simulink model "Modelo_final"  (R2020a)
settings: Solver=VariableStepAuto  StartTime=0.0  StopTime=20  RelTol=1e-3
values from neighbouring files (symbols this model uses):
  ba = Jeq*n*wpos    (= 0.0113019895361)    [Parametros.m]
  beq = bm+(bl/r^2)    (= 1.5e-05)    [Parametros.m]
  Cts = 1.091    [Parametros.m]
  Jeq = Jm+(Jl/r^2)    (= 5.65099476805e-06)    [Parametros.m]
  ke_omega = 3200^2    (= 10240000)    [Parametros.m]
  ke_thetha = 6400    [Parametros.m]
  ksa = Jeq*n*wpos^2    (= 9.04159162887)    [Parametros.m]
  ksia = Jeq*wpos^3    (= 2893.30932124)    [Parametros.m]
  lambdam = .01546    (= 0.01546)    [Parametros.m]
  Ld = 6.6e-3    (= 0.0066)    [Parametros.m]
  Lls = 0.8e-3    (= 0.0008)    [Parametros.m]
  Lq = 5.8e-3    (= 0.0058)    [Parametros.m]
  Pp = 3    [Parametros.m]
  r = 314.3008    [Parametros.m]
  R0p = 4    [Parametros.m]
  Rdp = 33    [Parametros.m]
  Rqp = 29    [Parametros.m]
  Rs = 1.02    [Parametros.m]
  Rs40 = 1.02    [Parametros.m]
  Rts = 55    [Parametros.m]
undefined symbols (not defined in the file or in its folder): sigbuilder_block
settings Model: Creator=tinsu  LastModifiedBy=tinsu

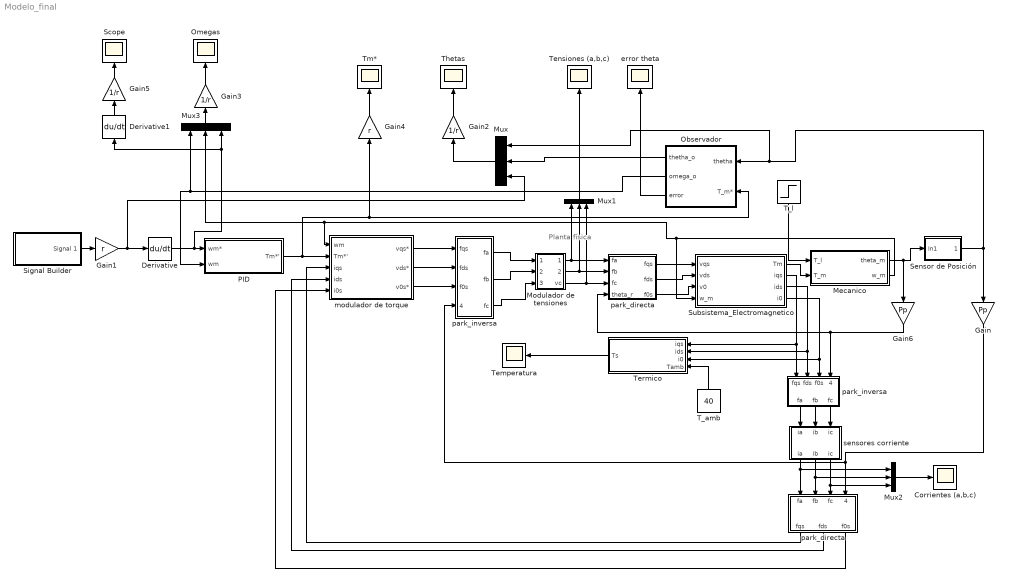
== system Modelo_final ==
  note: Planta física
  Corrientes (a,b,c) : Scope
  Derivative : Derivative
  Derivative1 : Derivative
  Gain : Gain  Gain=Pp
  Gain1 : Gain  Gain=r
  Gain2 : Gain  Gain=1/r
  Gain3 : Gain  Gain=1/r
  Gain4 : Gain  Gain=r
  Gain5 : Gain  Gain=1/r
  Gain6 : Gain  Gain=Pp
  Mecanico : Subsystem
  Modulador de tensiones : Subsystem
  Mux{,1..3} (4 alike) : Mux  Inputs=3
  Observador : Subsystem
  Omegas : Scope
  PID : Subsystem
  Scope : Scope
  Sensor de Posición : Subsystem
  Signal Builder : Subsystem  Tag=STV Subsys  LoadFcn=sigbuilder_block('load');  StartFcn=sigbuilder_block('start');  StopFcn=sigbuilder_block('stop');  ClipboardFcn=sigbuilder_block('clipboard');  mask(Sigbuilder block){tuvar=[0:10]}
      mask help: Simulink:masks:SigbuilderBlock_MD
      mask init:
      | if ~strcmp(get_param(bdroot(gcbh),'SimulationStatus'),'stopped') tuvar = sigbuilder_block('maskInit'); end
      settings: CopyFcn=sigbuilder_block('copy');  DeleteFcn=sigbuilder_block('delete');  ModelCloseFcn=sigbuilder_block('modelClose');  PreSaveFcn=sigbuilder_block('preSave');  PauseFcn=sigbuilder_block('pause');  ContinueFcn=sigbuilder_block('continue');  NameChangeFcn=sigbuilder_block('namechange');  OpenFcn=sigbuilder_block('open',[437.6 199.2 550.4 400 ]);  CloseFcn=sigbuilder_block('close');
      mask Display: plot(0, 0, 100, 100,[2, 2, 32, 32, 2], [68, 8, 8, 68, 68],[32, 2], [38, 38], [32, 19, 2],[53, 60, 44], [32, 17, 17, 2],[16, 16, 31, 31]);txt = getActiveGroup(gcbh);text(2, 100, txt,'verticalAlignment', 'top');
  Subsistema_Electromagnetico : Subsystem
  T_amb : Constant  Value=40
  T_l : Step  After=1.57  SampleTime=0
  Temperatura : Scope
  Tensiones (a,b,c) : Scope
  Termico : Subsystem
  Thetas : Scope
  Tm* : Scope
  error theta : Scope
  modulador de torque : Subsystem
  park_directa : Subsystem
  "park_directa " : Subsystem
  park_inversa : Subsystem
  "park_inversa " : Subsystem
  sensores corriente : Subsystem
  wires:
  Mux3/1 -> Gain3/1
  "park_directa "/2(fds) -> modulador de torque/4(ids)
  Gain3/1 -> Omegas/1
  Modulador de tensiones/1(va) -> Mux1/1, park_directa/1("fa ")
  Signal Builder/1(Signal 1) -> Gain1/1
  Gain4/1 -> Tm*/1
  Termico/1(Ts) -> Temperatura/1
  sensores corriente/1("ia ") -> "park_directa "/1("fa "), Mux2/1
  Observador/3(error) -> error theta/1
  Gain/1 -> "park_directa "/4(theta_r1), park_inversa/4(theta_r)
  "park_inversa "/1(fa) -> sensores corriente/1(ia)
  "park_directa "/1(fqs) -> modulador de torque/3(iqs)
  Mux1/1 -> Tensiones (a,b,c)/1
  Mux/1 -> Gain2/1
  Gain1/1 -> Derivative/1, Mux/3
  T_l/1 -> Mecanico/1(T_l)
  sensores corriente/2("ib ") -> "park_directa "/2("fb "), Mux2/2
  Mux2/1 -> Corrientes (a,b,c)/1
  park_directa/2(fds) -> Subsistema_Electromagnetico/2(vds)
  Gain2/1 -> Thetas/1
  Observador/1(thetha_o) -> Mux/2
  Mecanico/2(w_m) -> modulador de torque/1(wm), Mux3/2, Subsistema_Electromagnetico/4(w_m)
  park_directa/3(f0s) -> Subsistema_Electromagnetico/3(v0)
  Subsistema_Electromagnetico/2(iqs) -> Termico/1(iqs), "park_inversa "/1(fqs)
  Subsistema_Electromagnetico/3(ids) -> "park_inversa "/2(fds), Termico/2(ids)
  Observador/2(omega_o) -> Mux3/1, PID/2(wm)
  sensores corriente/3("ic ") -> Mux2/3, "park_directa "/3("fc ")
  Subsistema_Electromagnetico/4(i0) -> Termico/3(i0), "park_inversa "/3(f0s)
  Subsistema_Electromagnetico/1(Tm) -> Mecanico/2(T_m)
  "park_inversa "/2(fb) -> sensores corriente/2(ib)
  "park_inversa "/3(fc) -> sensores corriente/3(ic)
  Mecanico/1(theta_m) -> Gain6/1, Sensor de Posición/1(In1)
  modulador de torque/2(vds*) -> park_inversa/2(fds)
  PID/1(Tm*') -> Gain4/1, Observador/2(T_m*), modulador de torque/2(Tm*')
  park_inversa/1(fa) -> Modulador de tensiones/1(va*)
  park_inversa/3(fc) -> Modulador de tensiones/3(vc*)
  Modulador de tensiones/3(vc) -> Mux1/3, park_directa/3("fc ")
  "park_directa "/3(f0s) -> modulador de torque/5(i0s)
  modulador de torque/3(v0s*) -> park_inversa/3(f0s)
  park_inversa/2(fb) -> Modulador de tensiones/2(vb*)
  Modulador de tensiones/2(vb) -> Mux1/2, park_directa/2("fb ")
  modulador de torque/1(vqs*) -> park_inversa/1(fqs)
  T_amb/1 -> Termico/4(Tamb)
  park_directa/1(fqs) -> Subsistema_Electromagnetico/1(vqs)
  Derivative/1 -> Derivative1/1, Mux3/3, PID/1(wm*)
  Sensor de Posición/1(Out1) -> Gain/1, Mux/1, Observador/1(thetha)
  Derivative1/1 -> Gain5/1
  Gain5/1 -> Scope/1
  Gain6/1 -> "park_inversa "/4(theta_r), park_directa/4(theta_r)

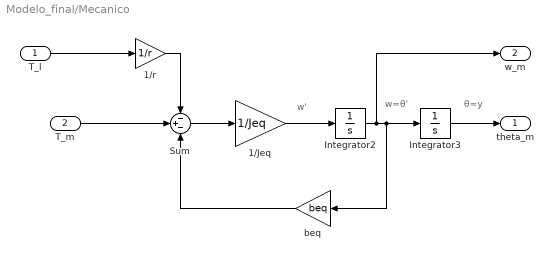
== system Modelo_final/Mecanico ==
  note: w=θ'
  note: θ=y
  note: w'
  T_l : Inport
  T_m : Inport  Port=2
  "1/Jeq " : Gain  Gain=1/Jeq
  "1/r " : Gain  Gain=1/r
  Integrator2 : Integrator
  Integrator3 : Integrator
  Sum : Sum  Inputs=-+-
  "beq " : Gain  Gain=beq
  theta_m : Outport
  w_m : Outport  Port=2
  wires:
  "1/r "/1 -> Sum/1
  "1/Jeq "/1 -> Integrator2/1
  Integrator3/1 -> theta_m/1
  Sum/1 -> "1/Jeq "/1
  "beq "/1 -> Sum/3
  Integrator2/1 -> Integrator3/1, "beq "/1, w_m/1
  T_m/1 -> Sum/2
  T_l/1 -> "1/r "/1

== system Modelo_final/Modulador de tensiones ==
  va* : Inport
  vb* : Inport  Port=2
  vc* : Inport  Port=3
  Gain : Gain
  Gain1 : Gain
  Gain2 : Gain
  va : Outport
  vb : Outport  Port=2
  vc : Outport  Port=3
  wires:
  va*/1 -> Gain/1
  vb*/1 -> Gain1/1
  vc*/1 -> Gain2/1
  Gain/1 -> va/1
  Gain1/1 -> vb/1
  Gain2/1 -> vc/1

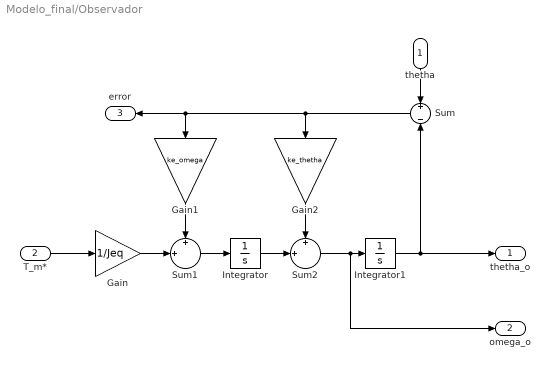
== system Modelo_final/Observador ==
  thetha : Inport
  T_m* : Inport  Port=2
  Gain : Gain  Gain=1/Jeq
  Gain1 : Gain  Gain=ke_omega
  Gain2 : Gain  Gain=ke_thetha
  Integrator : Integrator
  Integrator1 : Integrator
  Sum : Sum  Inputs=+||-
  Sum1 : Sum  Inputs=+|+||
  Sum2 : Sum  Inputs=+|+||
  thetha_o : Outport
  omega_o : Outport  Port=2
  error : Outport  Port=3
  wires:
  Integrator1/1 -> thetha_o/1, Sum/2
  T_m*/1 -> Gain/1
  Sum/1 -> error/1, Gain1/1, Gain2/1
  Gain1/1 -> Sum1/1
  thetha/1 -> Sum/1
  Integrator/1 -> Sum2/2
  Sum1/1 -> Integrator/1
  Gain2/1 -> Sum2/1
  Gain/1 -> Sum1/2
  Sum2/1 -> omega_o/1, Integrator1/1

== system Modelo_final/PID ==
  note: I
  note: e_dtheta_m
  note: e_wm
  note: e_theta_m
  note: P
  note: D
  wm* : Inport
  wm : Inport  Port=2
  Integrator : Integrator
  Integrator1 : Integrator
  Sum : Sum  Inputs=|+-
  Sum1 : Sum  Inputs=|+++
  ba : Gain  Gain=ba
  ksa : Gain  Gain=ksa
  ksia : Gain  Gain=ksia
  Tm*' : Outport
  wires:
  Integrator1/1 -> ksia/1
  Sum1/1 -> Tm*'/1
  wm*/1 -> Sum/1
  ba/1 -> Sum1/3
  Sum/1 -> Integrator/1, ba/1
  ksa/1 -> Sum1/2
  ksia/1 -> Sum1/1
  wm/1 -> Sum/2
  Integrator/1 -> Integrator1/1, ksa/1

== system Modelo_final/Sensor de Posición ==
  In1 : Inport
  Gain : Gain
  Out1 : Outport
  wires:
  In1/1 -> Gain/1
  Gain/1 -> Out1/1

== system Modelo_final/Signal Builder ==
  Demux : Demux  Tag=STV Demux  Outputs=1
      settings: DisplayOption=none
  FromWs : FromWorkspace  Tag=STV FromWs  VariableName=tuvar
      SigBuilderData=|
      | common.afterFinalStr = 'Extrapolate'
      | common.sampleTime = 0
      | dataSet.timeRange = [0 20]
      | dataSet.name = 'Group 1'
      | sbobj.Groups.Name = 'Group 1'
      | sbobj.Groups.Signals.Name = 'Signal 1'
      | sbobj.Groups.Signals.XData = [0 2 7 13 18 20]
      | sbobj.Groups.Signals.YData = [0 0 6.28318530718 6.28318530718 0 0]
      | sbobj.Groups.TimeRange = [0 20]
  Signal 1 : Outport  Tag=STV Outport
  wires:
  Demux/1 -> Signal 1/1
  FromWs/1 -> Demux/1

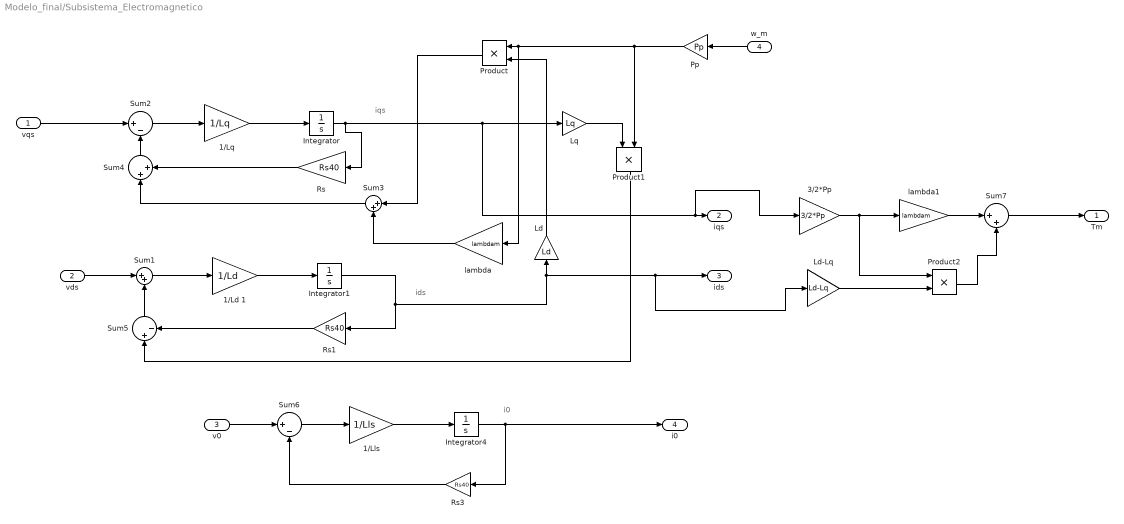
== system Modelo_final/Subsistema_Electromagnetico ==
  note: iqs
  note: i0
  note: ids
  vqs : Inport
  vds : Inport  Port=2
  v0 : Inport  Port=3
  w_m : Inport  Port=4
  1/Ld 1 : Gain  Gain=1/Ld
  1/Lls : Gain  Gain=1/Lls
  "1/Lq " : Gain  Gain=1/Lq
  3/2*Pp : Gain  Gain=3/2*Pp
  Integrator : Integrator
  Integrator1 : Integrator
  Integrator4 : Integrator
  Ld : Gain  Gain=Ld
  Ld-Lq : Gain  Gain=Ld-Lq
  "Lq " : Gain  Gain=Lq
  Pp : Gain  Gain=Pp
  Product : Product
  Product1 : Product
  Product2 : Product
  Rs : Gain  Gain=Rs40
  Rs1 : Gain  Gain=Rs40
  Rs3 : Gain  Gain=Rs40
  Sum{1,3..4,7} (4 alike) : Sum  Inputs=|++
  Sum2 : Sum  Inputs=|+-
  Sum5 : Sum  Inputs=|+-
  Sum6 : Sum  Inputs=|+-
  lambda : Gain  Gain=lambdam
  lambda1 : Gain  Gain=lambdam
  Tm : Outport
  iqs : Outport  Port=2
  ids : Outport  Port=3
  i0 : Outport  Port=4
  wires:
  Integrator4/1 -> i0/1, Rs3/1
  Sum6/1 -> 1/Lls/1
  Sum5/1 -> Sum1/2
  Rs/1 -> Sum4/2
  Sum4/1 -> Sum2/2
  "1/Lq "/1 -> Integrator/1
  Integrator1/1 -> Rs1/1, Ld-Lq/1, ids/1, Ld/1
  Integrator/1 -> Rs/1, 3/2*Pp/1, iqs/1, "Lq "/1
  Rs3/1 -> Sum6/2
  1/Lls/1 -> Integrator4/1
  Product/1 -> Sum3/1
  Pp/1 -> lambda/1, Product/1, Product1/2
  "Lq "/1 -> Product1/1
  Sum1/1 -> 1/Ld 1/1
  Product1/1 -> Sum5/1
  1/Ld 1/1 -> Integrator1/1
  Sum2/1 -> "1/Lq "/1
  v0/1 -> Sum6/1
  lambda/1 -> Sum3/2
  Ld/1 -> Product/2
  Rs1/1 -> Sum5/2
  vds/1 -> Sum1/1
  Sum3/1 -> Sum4/1
  vqs/1 -> Sum2/1
  w_m/1 -> Pp/1
  Ld-Lq/1 -> Product2/2
  lambda1/1 -> Sum7/1
  Product2/1 -> Sum7/2
  3/2*Pp/1 -> Product2/1, lambda1/1
  Sum7/1 -> Tm/1

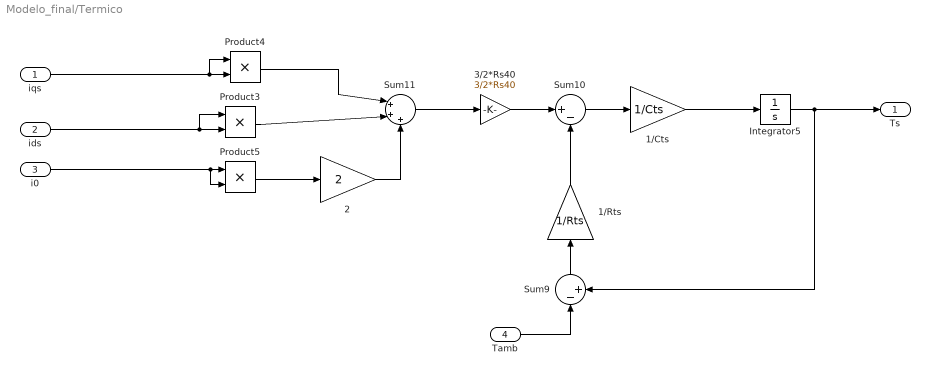
== system Modelo_final/Termico ==
  iqs : Inport
  ids : Inport  Port=2
  i0 : Inport  Port=3
  Tamb : Inport  Port=4
  1/Cts : Gain  Gain=1/Cts
  1/Rts : Gain  Gain=1/Rts
  "2 " : Gain  Gain=2
  "3/2*Rs40 " : Gain  Gain=3/2*Rs40
  Integrator5 : Integrator
  Product3 : Product
  Product4 : Product
  Product5 : Product
  Sum10 : Sum  Inputs=|+-
  Sum11 : Sum  Inputs=|+++
  Sum9 : Sum  Inputs=|-+
  Ts : Outport
  wires:
  "3/2*Rs40 "/1 -> Sum10/1
  1/Cts/1 -> Integrator5/1
  Sum10/1 -> 1/Cts/1
  Tamb/1 -> Sum9/1
  Integrator5/1 -> Ts/1, Sum9/2
  Product3/1 -> Sum11/2
  ids/1 -> Product3/1, Product3/2
  "2 "/1 -> Sum11/3
  Sum11/1 -> "3/2*Rs40 "/1
  Product5/1 -> "2 "/1
  i0/1 -> Product5/2, Product5/1
  1/Rts/1 -> Sum10/2
  Product4/1 -> Sum11/1
  Sum9/1 -> 1/Rts/1
  iqs/1 -> Product4/1, Product4/2

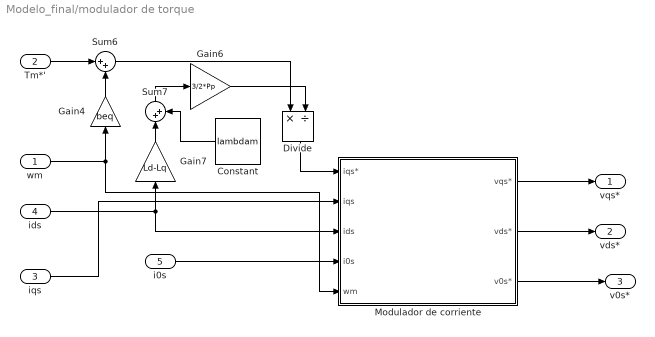
== system Modelo_final/modulador de torque ==
  wm : Inport
  Tm*' : Inport  Port=2
  iqs : Inport  Port=3
  ids : Inport  Port=4
  i0s : Inport  Port=5
  Constant : Constant  Value=lambdam
  Divide : Product  Inputs=*/
  Gain4 : Gain  Gain=beq
  Gain6 : Gain  Gain=3/2*Pp
  Gain7 : Gain  Gain=Ld-Lq
  Modulador de corriente : Subsystem
  Sum6 : Sum  Inputs=|++
  Sum7 : Sum  Inputs=|++
  vqs* : Outport
  vds* : Outport  Port=2
  v0s* : Outport  Port=3
  wires:
  iqs/1 -> Modulador de corriente/2(iqs)
  ids/1 -> Modulador de corriente/3(ids), Gain7/1
  Modulador de corriente/2(vds*) -> vds*/1
  Modulador de corriente/1(vqs*) -> vqs*/1
  Gain7/1 -> Sum7/1
  i0s/1 -> Modulador de corriente/4(i0s)
  Gain6/1 -> Divide/2
  Divide/1 -> Modulador de corriente/1(iqs*)
  wm/1 -> Modulador de corriente/5(wm), Gain4/1
  Gain4/1 -> Sum6/2
  Constant/1 -> Sum7/2
  Tm*'/1 -> Sum6/1
  Sum7/1 -> Gain6/1
  Sum6/1 -> Divide/1
  Modulador de corriente/3(v0s*) -> v0s*/1

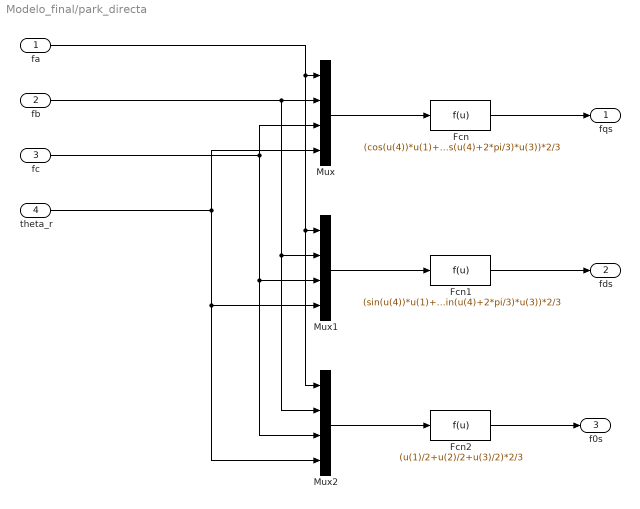
== system Modelo_final/park_directa ==
  "fa " : Inport
  "fb " : Inport  Port=2
  "fc " : Inport  Port=3
  theta_r : Inport  Port=4
  Fcn : Fcn  Expr=(cos(u(4))*u(1)+cos(u(4)-2*pi/3)*u(2)+cos(u(4)+2*pi/3)*u(3))*2/3
  Fcn1 : Fcn  Expr=(sin(u(4))*u(1)+sin(u(4)-2*pi/3)*u(2)+sin(u(4)+2*pi/3)*u(3))*2/3
  Fcn2 : Fcn  Expr=(u(1)/2+u(2)/2+u(3)/2)*2/3
  Mux : Mux
  Mux1 : Mux
  Mux2 : Mux
  fqs : Outport
  fds : Outport  Port=2
  f0s : Outport  Port=3
  wires:
  "fc "/1 -> Mux/3, Mux1/3, Mux2/3
  "fb "/1 -> Mux/2, Mux1/2, Mux2/2
  Fcn/1 -> fqs/1
  Fcn2/1 -> f0s/1
  theta_r/1 -> Mux/4, Mux1/4, Mux2/4
  Mux2/1 -> Fcn2/1
  Mux1/1 -> Fcn1/1
  Mux/1 -> Fcn/1
  Fcn1/1 -> fds/1
  "fa "/1 -> Mux1/1, Mux2/1, Mux/1

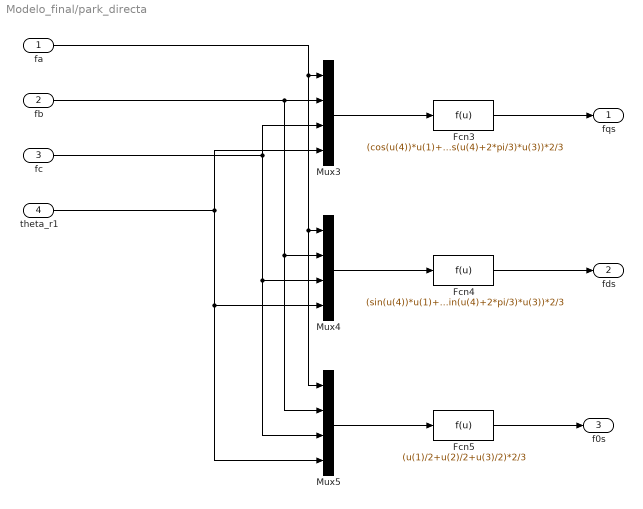
== system Modelo_final/park_directa  ==
  "fa " : Inport
  "fb " : Inport  Port=2
  "fc " : Inport  Port=3
  theta_r1 : Inport  Port=4
  Fcn3 : Fcn  Expr=(cos(u(4))*u(1)+cos(u(4)-2*pi/3)*u(2)+cos(u(4)+2*pi/3)*u(3))*2/3
  Fcn4 : Fcn  Expr=(sin(u(4))*u(1)+sin(u(4)-2*pi/3)*u(2)+sin(u(4)+2*pi/3)*u(3))*2/3
  Fcn5 : Fcn  Expr=(u(1)/2+u(2)/2+u(3)/2)*2/3
  Mux3 : Mux
  Mux4 : Mux
  Mux5 : Mux
  fqs : Outport
  fds : Outport  Port=2
  f0s : Outport  Port=3
  wires:
  Mux5/1 -> Fcn5/1
  "fa "/1 -> Mux4/1, Mux5/1, Mux3/1
  Fcn4/1 -> fds/1
  Mux3/1 -> Fcn3/1
  Mux4/1 -> Fcn4/1
  "fb "/1 -> Mux3/2, Mux4/2, Mux5/2
  Fcn3/1 -> fqs/1
  Fcn5/1 -> f0s/1
  theta_r1/1 -> Mux3/4, Mux4/4, Mux5/4
  "fc "/1 -> Mux3/3, Mux4/3, Mux5/3

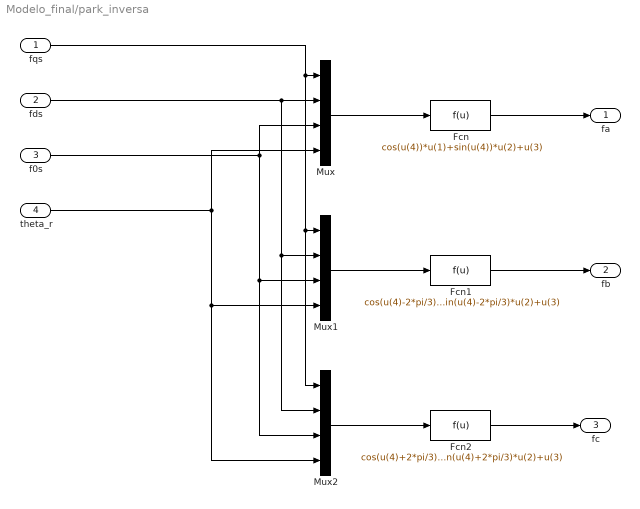
== system Modelo_final/park_inversa ==
  fqs : Inport
  fds : Inport  Port=2
  f0s : Inport  Port=3
  theta_r : Inport  Port=4
  Fcn : Fcn  Expr=cos(u(4))*u(1)+sin(u(4))*u(2)+u(3)
  Fcn1 : Fcn  Expr=cos(u(4)-2*pi/3)*u(1)+sin(u(4)-2*pi/3)*u(2)+u(3)
  Fcn2 : Fcn  Expr=cos(u(4)+2*pi/3)*u(1)+sin(u(4)+2*pi/3)*u(2)+u(3)
  Mux : Mux
  Mux1 : Mux
  Mux2 : Mux
  fa : Outport
  fb : Outport  Port=2
  fc : Outport  Port=3
  wires:
  f0s/1 -> Mux/3, Mux1/3, Mux2/3
  fds/1 -> Mux/2, Mux1/2, Mux2/2
  Fcn/1 -> fa/1
  Fcn2/1 -> fc/1
  theta_r/1 -> Mux/4, Mux1/4, Mux2/4
  Mux2/1 -> Fcn2/1
  Mux1/1 -> Fcn1/1
  Mux/1 -> Fcn/1
  Fcn1/1 -> fb/1
  fqs/1 -> Mux1/1, Mux2/1, Mux/1

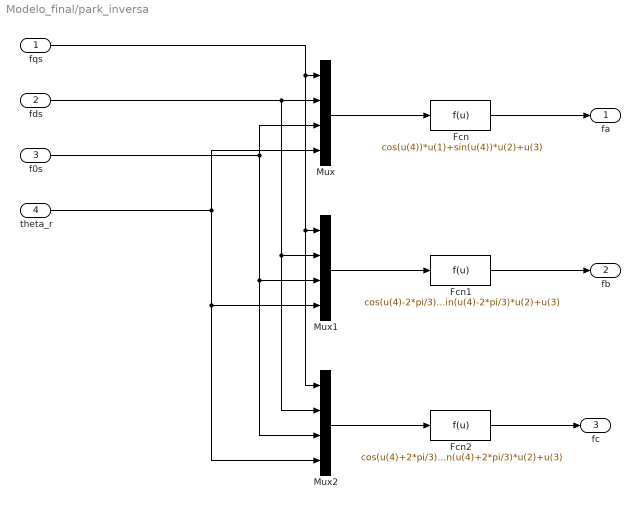
== system Modelo_final/park_inversa  ==
  fqs : Inport
  fds : Inport  Port=2
  f0s : Inport  Port=3
  theta_r : Inport  Port=4
  Fcn : Fcn  Expr=cos(u(4))*u(1)+sin(u(4))*u(2)+u(3)
  Fcn1 : Fcn  Expr=cos(u(4)-2*pi/3)*u(1)+sin(u(4)-2*pi/3)*u(2)+u(3)
  Fcn2 : Fcn  Expr=cos(u(4)+2*pi/3)*u(1)+sin(u(4)+2*pi/3)*u(2)+u(3)
  Mux : Mux
  Mux1 : Mux
  Mux2 : Mux
  fa : Outport
  fb : Outport  Port=2
  fc : Outport  Port=3
  wires:
  f0s/1 -> Mux/3, Mux1/3, Mux2/3
  fds/1 -> Mux/2, Mux1/2, Mux2/2
  Fcn/1 -> fa/1
  Fcn2/1 -> fc/1
  theta_r/1 -> Mux/4, Mux1/4, Mux2/4
  Mux2/1 -> Fcn2/1
  Mux1/1 -> Fcn1/1
  Mux/1 -> Fcn/1
  Fcn1/1 -> fb/1
  fqs/1 -> Mux1/1, Mux2/1, Mux/1

== system Modelo_final/sensores corriente ==
  ia : Inport
  ib : Inport  Port=2
  ic : Inport  Port=3
  Gain : Gain
  Gain1 : Gain
  Gain2 : Gain
  "ia " : Outport
  "ib " : Outport  Port=2
  "ic " : Outport  Port=3
  wires:
  ia/1 -> Gain/1
  ib/1 -> Gain1/1
  ic/1 -> Gain2/1
  Gain/1 -> "ia "/1
  Gain1/1 -> "ib "/1
  Gain2/1 -> "ic "/1

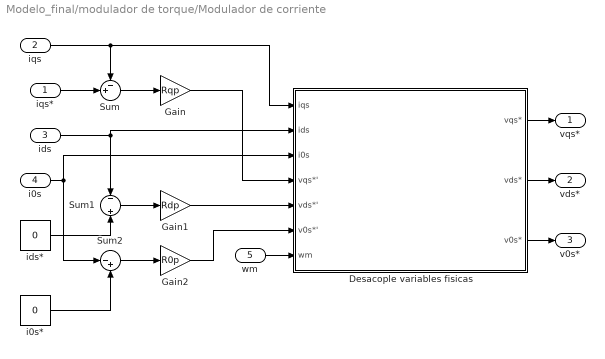
== system Modelo_final/modulador de torque/Modulador de corriente ==
  iqs* : Inport
  iqs : Inport  Port=2
  ids : Inport  Port=3
  i0s : Inport  Port=4
  wm : Inport  Port=5
  Desacople variables fisicas : Subsystem
  Gain : Gain  Gain=Rqp
  Gain1 : Gain  Gain=Rdp
  Gain2 : Gain  Gain=R0p
  Sum : Sum  Inputs=-+|
  Sum1 : Sum  Inputs=-||+
  Sum2 : Sum  Inputs=|-+
  i0s* : Constant  Value=0
  ids* : Constant  Value=0
  vqs* : Outport
  vds* : Outport  Port=2
  v0s* : Outport  Port=3
  wires:
  Sum/1 -> Gain/1
  Gain/1 -> Desacople variables fisicas/4(vqs*')
  Desacople variables fisicas/1(vqs*) -> vqs*/1
  Gain2/1 -> Desacople variables fisicas/6(v0s*')
  wm/1 -> Desacople variables fisicas/7(wm)
  Desacople variables fisicas/3(v0s*) -> v0s*/1
  i0s*/1 -> Sum2/2
  iqs*/1 -> Sum/2
  ids*/1 -> Sum1/2
  Desacople variables fisicas/2(vds*) -> vds*/1
  Sum1/1 -> Gain1/1
  iqs/1 -> Sum/1, Desacople variables fisicas/1(iqs)
  Sum2/1 -> Gain2/1
  i0s/1 -> Desacople variables fisicas/3(i0s), Sum2/1
  Gain1/1 -> Desacople variables fisicas/5(vds*')
  ids/1 -> Desacople variables fisicas/2(ids), Sum1/1

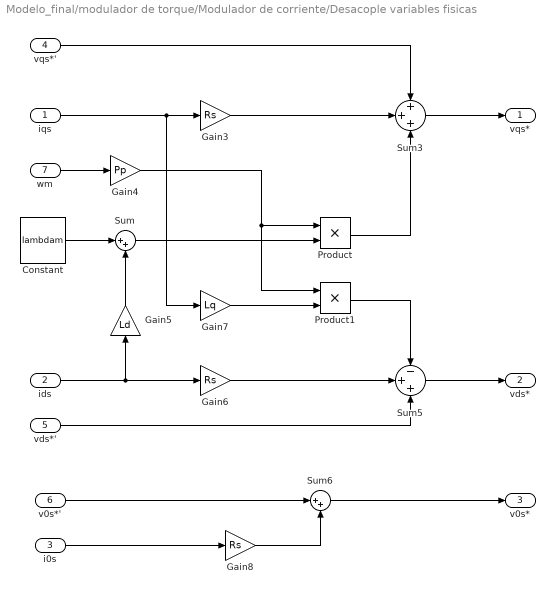
== system Modelo_final/modulador de torque/Modulador de corriente/Desacople variables fisicas ==
  iqs : Inport
  ids : Inport  Port=2
  i0s : Inport  Port=3
  vqs*' : Inport  Port=4
  vds*' : Inport  Port=5
  v0s*' : Inport  Port=6
  wm : Inport  Port=7
  Constant : Constant  Value=lambdam
  Gain3 : Gain  Gain=Rs
  Gain4 : Gain  Gain=Pp
  Gain5 : Gain  Gain=Ld
  Gain6 : Gain  Gain=Rs
  Gain7 : Gain  Gain=Lq
  Gain8 : Gain  Gain=Rs
  Product : Product
  Product1 : Product
  Sum : Sum  Inputs=|++
  Sum3 : Sum  Inputs=+++
  Sum5 : Sum  Inputs=-++
  Sum6 : Sum  Inputs=|++
  vqs* : Outport
  vds* : Outport  Port=2
  v0s* : Outport  Port=3
  wires:
  Gain5/1 -> Sum/2
  Constant/1 -> Sum/1
  Gain7/1 -> Product1/2
  vqs*'/1 -> Sum3/1
  vds*'/1 -> Sum5/3
  Gain8/1 -> Sum6/2
  i0s/1 -> Gain8/1
  Sum/1 -> Product/2
  v0s*'/1 -> Sum6/1
  iqs/1 -> Gain3/1, Gain7/1
  Sum6/1 -> v0s*/1
  Gain6/1 -> Sum5/2
  Sum5/1 -> vds*/1
  Product1/1 -> Sum5/1
  Gain3/1 -> Sum3/2
  ids/1 -> Gain6/1, Gain5/1
  Product/1 -> Sum3/3
  Sum3/1 -> vqs*/1
  Gain4/1 -> Product1/1, Product/1
  wm/1 -> Gain4/1
